simulink model "Battery_Harness"  (R2025a)
settings: Solver=FixedStepAuto  StartTime=0.0  StopTime=10  RelTol=1e-3
libraries: fl_lib x1, nesl_utility x1, ee_lib x1
settings Model: Creator=skota  LastModifiedBy=skota
settings GRTTargetCC: UtilityFuncGeneration=Shared location

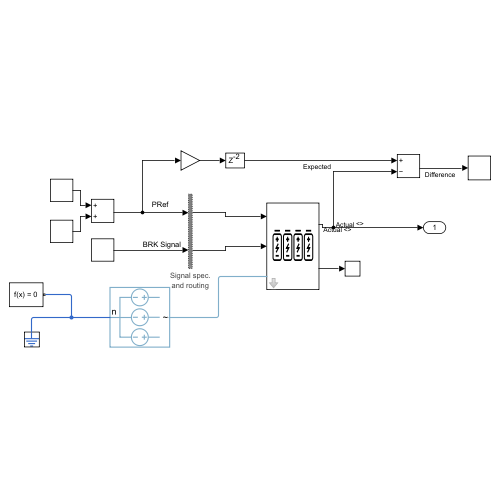
[thumbnail: Simulink's stored preview of the top-level diagram]
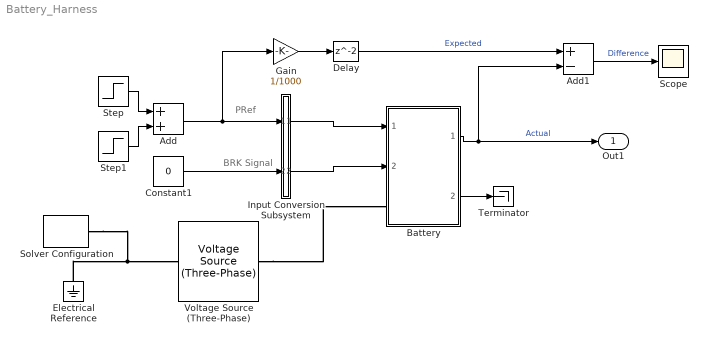
== system Battery_Harness ==
  note: PRef
  note: BRK Signal
  Add : Sum
  Add1 : Sum  Inputs=+-
  Battery : Subsystem  ReferencedSubsystem=Battery  minSOC=0  maxSOC=1  energyRating=100  capacityRating=40.77  nominalVoltage=1280  frequency=60  windingRatio=1
  Constant1 : Constant  Value=0  OutDataTypeStr=boolean
  Delay : Delay
  Electrical Reference : fl_lib/Electrical/Electrical Elements/Electrical Reference
  Gain : Gain  Gain=1/1000
  Input Conversion Subsystem : Subsystem  Tag=__SLT_ICS__  Description=|
      | Signal spec.
      | and routing
      settings: AttributesFormatString=%<Description>
  Scope : Scope
      settings: ActiveDisplayYMinimum=-2.17273  ActiveDisplayYMaximum=11.46362  DataLoggingVariableName=ScopeData2
  Solver Configuration : nesl_utility/Solver Configuration  PhysicalDomain=network_engine_domain  SubClassName=solver  LeftPortType=input  RightPortType=generic  Tones=[]  Harmonics=[]  SimulateNoise=off  Profile=off  UseLocalSampling=off  EnableSwitchedLinearOptims=on  FrequencyDomain=off  UseCCode=off  RelTol=0.001  AbsTol=0.001  MinStep=1e-09  ToWorkspace=off  RevertToSquareIcSolve=off  NumHomotopyIterations=100  PhasorMode=off  PhasorModeNumHarmonics=1  ConsistencySolver=NEWTON_XTOL_AFTER_FTOL  IndexReductionMethod=DerivativeReplacement  DoDC=off  ResidualTolerance=1e-09  ConsistencyTolSource=GLOBAL  ConsistencyAbsTol=0.001  ConsistencyRelTol=0.001  ConsistencyTolFactor=0.001  UseLocalSolver=on  LocalSolverChoice=NE_BACKWARD_EULER_ADVANCER  ResolveIndetEquations=on  FunctionEvalNumThread=1  LocalSolverSampleTime=0.001  DoFixedCost=on  MaxNonlinIter=3  MaxModeIter=2  ComputeImpulses=off  ImpulseIterations=2  LinearAlgebra=auto  LinearAlgebraNumThread=0  EquationFormulation=NE_FREQUENCY_TIME_EF  DelaysMemoryBudget=1024  AutomaticFiltering=on  FilteringTimeConstant=0.001  PartitionStorageMethod=AS_NEEDED  PartitionMemoryBudget=1024  PartitionMethod=ROBUST  MultibodyUseLocalSolver=off  MultibodyLocalSolverChoice=ODE1  MultibodyLocalSolverSampleTime=0.001
  Step : Step  Time=0  After=5000  SampleTime=0
  Step1 : Step  Time=5  After=-10000  SampleTime=0
  Terminator : Terminator
  Voltage Source (Three-Phase) : ee_lib/Sources/Voltage Source (Three-Phase)  vline_rms=1000 V  shift=0 deg  freq=60 Hz  impedance_option=0  SShortCircuit=1e6 A*V  XR=15  R=0.01 Ohm  L=3.97e-4 H  harmonic_option=0  harmonic_orders=[5, 7, 11, 13]  harmonic_ratios=[.1, .1, .1, .1]  G_parasitic=0 1/Ohm  I_specify=off  I_priority=None  I=[0, 0, 0] A  I_nominal_specify=off  I_nominal_value=1  I_nominal_unit=A
  Out1 : Outport
  wires:
  Constant1/1 -> Input Conversion Subsystem/2(Inport_2)
  Battery/1 -> Add1/2, Out1/1  "Actual"
  Input Conversion Subsystem/1(Outport_1) -> Battery/1
  Input Conversion Subsystem/2(Outport_2) -> Battery/2
  Step/1 -> Add/1
  Step1/1 -> Add/2
  Add/1 -> Gain/1, Input Conversion Subsystem/1(Inport_1)
  Add1/1 -> Scope/1  "Difference"
  Delay/1 -> Add1/1  "Expected"
  Gain/1 -> Delay/1
  Battery/2 -> Terminator/1
  connections:
  Voltage Source (Three-Phase)/RConn1 -- Battery/LConn1
  Electrical Reference/LConn1 -- Solver Configuration/RConn1 -- Voltage Source (Three-Phase)/LConn1

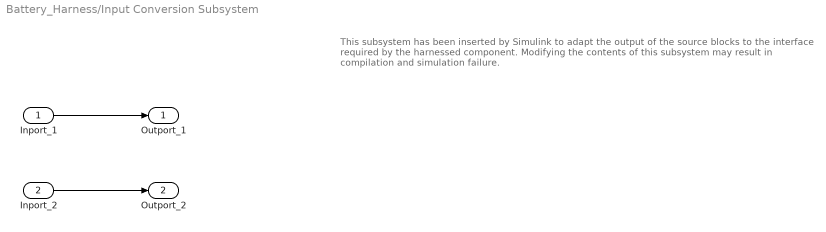
== system Battery_Harness/Input Conversion Subsystem ==
  note: This subsystem has been inserted by Simulink to adapt the output of the source blocks to the interface required by the harnessed component.
      |  Modifying the contents of this subsystem may result in compilation and simulation failure.
  Inport_1 : Inport
  Inport_2 : Inport  Port=2
  Outport_1 : Outport
  Outport_2 : Outport  Port=2
  wires:
  Inport_1/1 -> Outport_1/1
  Inport_2/1 -> Outport_2/1
